simulink model "generalizedPlant"  (R2019a)
settings: Solver=VariableStepAuto  StartTime=0.0  StopTime=10.0  RelTol=1e-3  EnableMultiTasking=on
undefined symbols (not defined in the file): nzKS, nzS
libraries: cstblocks x3
settings Model: Creator=chris  LastModifiedBy=Marlin Siebert
settings DataIOCC: ReturnWorkspaceOutputs=off
settings OptimizationCC: LifeSpan=inf
settings DebuggingCC: SFUnexpectedBacktrackingDiag=warning  SFNoUnconditionalDefaultTransitionDiag=warning  SFExecutionAtInitializationDiag=none  ArithmeticOperatorsInVariantConditions=warning
settings SFSimCC: SimUseLocalCustomCode=off
settings RTWCC: RTWUseLocalCustomCode=off
settings CodeAppCC: StateflowObjectComments=on
settings GRTTargetCC: TargetLangStandard=C89/C90 (ANSI)  GeneratePreprocessorConditionals=Disable all
settings ConfigComp: CovMetricSettings=dw  CovHtmlReporting=on  CovSaveCumulativeToWorkspaceVar=on  CovSaveSingleToWorkspaceVar=on  CovExternalEMLEnable=off

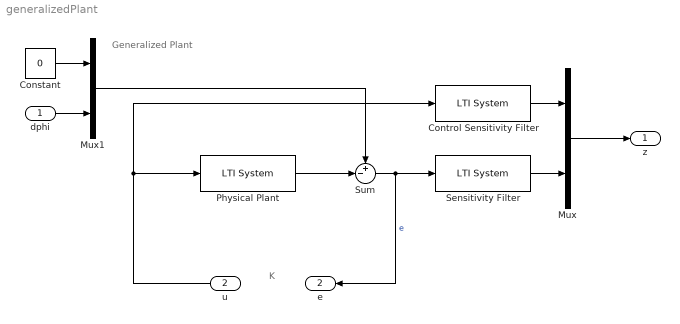
== system generalizedPlant ==
  note: K
  note: Generalized Plant
  dphi : Inport
  u : Inport  Port=2
  Constant : Constant  Value=0
  Control Sensitivity Filter : cstblocks/LTI System  sys=WKS  IC=[]
  Mux : Mux  Inputs=[nzKS, nzS]
  Mux1 : Mux  Inputs=2
  Physical Plant : cstblocks/LTI System  sys=G_gen_0  IC=[]
  Sensitivity Filter : cstblocks/LTI System  sys=WS  IC=[]
  Sum : Sum  Inputs=+-|
  z : Outport
  e : Outport  Port=2
  wires:
  u/1 -> Control Sensitivity Filter/1, Physical Plant/1
  Physical Plant/1 -> Sum/2
  Sum/1 -> Sensitivity Filter/1, e/1  "e"
  Control Sensitivity Filter/1 -> Mux/1
  Sensitivity Filter/1 -> Mux/2
  Mux/1 -> z/1
  Constant/1 -> Mux1/1
  dphi/1 -> Mux1/2
  Mux1/1 -> Sum/1
